simulink model "run_example"  (R2024a)
settings: Solver=FixedStepAuto  StartTime=0.0  StopTime=10.0  FixedStep=0.001  RelTol=1e-3
libraries: simulink x2
settings Model: Creator=autod  LastModifiedBy=autod
settings DebuggingCC: UnderspecifiedInitializationDetection=Classic  FrameProcessingCompatibilityMsg=none

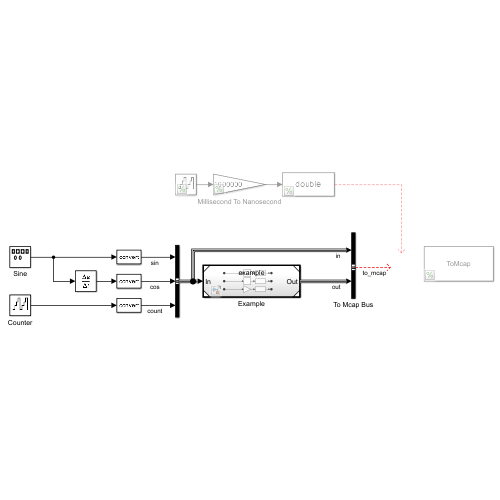
[thumbnail: Simulink's stored preview of the top-level diagram]
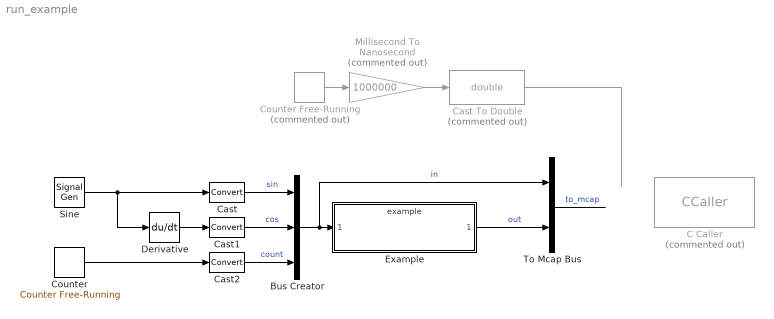
== system run_example ==
  Bus Creator : BusCreator  Inputs=3
  C Caller : CCaller  Commented=on  FunctionName=ToMcap
  Cast : DataTypeConversion  SaturateOnIntegerOverflow=off  RndMeth=Floor
  Cast To Double : DataTypeConversion  Commented=on  OutDataTypeStr=double  SaturateOnIntegerOverflow=off  RndMeth=Floor
  Cast1 : DataTypeConversion  SaturateOnIntegerOverflow=off  RndMeth=Floor
  Cast2 : DataTypeConversion  SaturateOnIntegerOverflow=off  RndMeth=Floor
  Counter : simulink/Sources/Counter Free-Running  NumBits=64  tsamp=-1
  Counter Free-Running : simulink/Sources/Counter Free-Running  Commented=on  NumBits=64  tsamp=-1
  Derivative : Derivative
  Example : ModelReference  ModelNameDialog=example.slx  SimulationMode=Normal  ModelReferenceVersion=4.64
  Millisecond To Nanosecond : Gain  Commented=on  Gain=1000000  OutDataTypeStr=uint64
  Sine : SignalGenerator  Units=rad/sec
  To Mcap Bus : BusCreator  Inputs=2
  wires:
  Example/1 -> To Mcap Bus/2  "out"
  Cast To Double/1 -> ?
  Counter Free-Running/1 -> Millisecond To Nanosecond/1
  Millisecond To Nanosecond/1 -> Cast To Double/1
  Sine/1 -> Derivative/1, Cast/1
  Derivative/1 -> Cast1/1
  Bus Creator/1 -> To Mcap Bus/1, Example/1  "in"
  Counter/1 -> Cast2/1
  Cast/1 -> Bus Creator/1  "sin"
  Cast1/1 -> Bus Creator/2  "cos"
  Cast2/1 -> Bus Creator/3  "count"
  To Mcap Bus/1 -> ?  "to_mcap"
